simulink model "controller_final"  (R2024a)
settings: Solver=FixedStepAuto  StartTime=0.0  StopTime=10.0  FixedStep=1/100  RelTol=1e-3
settings Model: Creator=DAUIN-Win10  LastModifiedBy=mahdy
settings OptimizationCC: ReuseModelBlockBuffer=off
settings DebuggingCC: UnconnectedInputMsg=warning  UnconnectedOutputMsg=warning  UnconnectedLineMsg=warning
settings ModelReferenceCC: EnableRefExpFcnMdlSchedulingChecks=on
settings RTWCC: GPUComputeCapability=3.5  DLArmComputeVersion=19.05

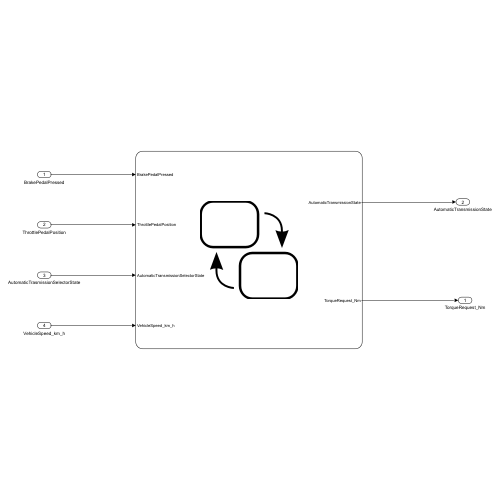
[thumbnail: Simulink's stored preview of the top-level diagram]
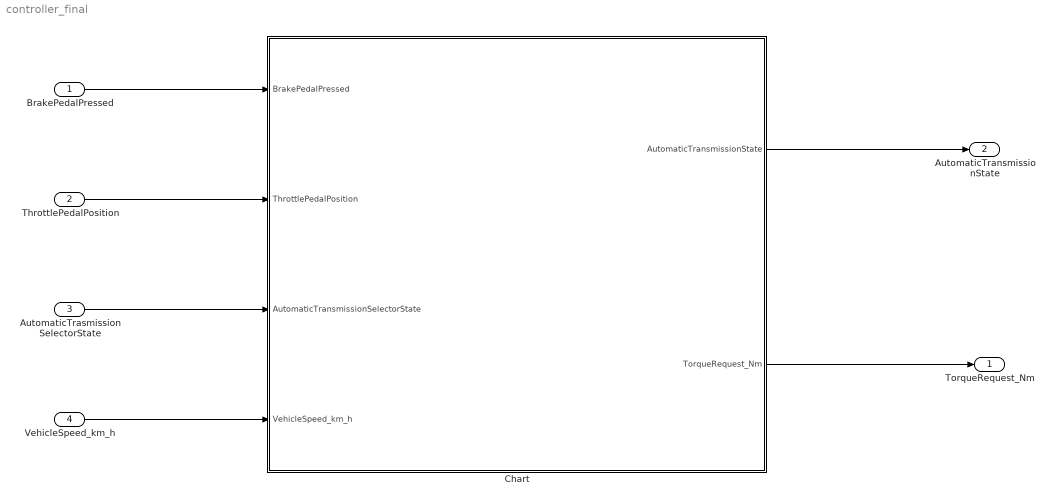
== system controller_final ==
  BrakePedalPressed : Inport  OutDataTypeStr=boolean
  ThrottlePedalPosition : Inport  Port=2  OutDataTypeStr=single
  AutomaticTrasmissionSelectorState : Inport  Port=3  OutDataTypeStr=Enum: TransmissionState
  VehicleSpeed_km_h : Inport  Port=4  OutDataTypeStr=single  Unit=km/h
  Chart : Stateflow chart  TreatAsAtomicUnit=on
  TorqueRequest_Nm : Outport  OutDataTypeStr=single  Unit=N*m
  AutomaticTransmissionState : Outport  Port=2  OutDataTypeStr=Enum: TransmissionState
  wires:
  VehicleSpeed_km_h/1 -> Chart/4(VehicleSpeed_km_h)
  AutomaticTrasmissionSelectorState/1 -> Chart/3(AutomaticTransmissionSelectorState)
  ThrottlePedalPosition/1 -> Chart/2(ThrottlePedalPosition)
  BrakePedalPressed/1 -> Chart/1(BrakePedalPressed)
  Chart/1(AutomaticTransmissionState) -> AutomaticTransmissionState/1
  Chart/2(TorqueRequest_Nm) -> TorqueRequest_Nm/1

== stateflow chart controller_final/Chart ==
  state Reverse
    entry:
    AutomaticTransmissionState =TransmissionState. Reverse;
    during:
    TorqueRequest_Nm = -ThrottlePedalPosition*MAX_TORQUE_REVERSE;
  state Park
    entry:
    AutomaticTransmissionState = TransmissionState.Park;
    TorqueRequest_Nm = 0;
  state Neutral
    entry:
    AutomaticTransmissionState = TransmissionState.Neutral;
    TorqueRequest_Nm = 0;
  state Bmode
    entry:
    AutomaticTransmissionState = TransmissionState.Brake;
    state Regenerative_Braking
      during:
      TorqueRequest_Nm =- MAX_TORQUE*(1-3*ThrottlePedalPosition)
    state Acceleration
      during:
      TorqueRequest_Nm =MAX_TORQUE*(ThrottlePedalPosition-1/3)*3/2;
    state Stop
      entry:
      TorqueRequest_Nm = 0;
    Acceleration -> Regenerative_Braking : [ThrottlePedalPosition<=1/3]
    Regenerative_Braking -> Acceleration [order 1] : [ThrottlePedalPosition>1/3]
    Stop -> Acceleration : [ThrottlePedalPosition>1/3]
    Regenerative_Braking -> Stop [order 2] : [ 0<ThrottlePedalPosition<=1/3 &&VehicleSpeed_km_h<=0.05 ]
    (default) -> Stop
  state Drive
    entry:
    AutomaticTransmissionState = TransmissionState.Drive;
    during:
    TorqueRequest_Nm = ThrottlePedalPosition*MAX_TORQUE;
  Reverse -> Neutral : [AutomaticTransmissionSelectorState ==TransmissionState. Neutral || AutomaticTransmissionSelectorState ==TransmissionState. Drive ||AutomaticTransmissionSelectorState ==TransmissionState. Brake||AutomaticTransmissionSelectorState ==TransmissionState. Park]
  Neutral -> Reverse [order 3] : [ VehicleSpeed_km_h<5 && AutomaticTransmissionSelectorState ==TransmissionState. Reverse &&BrakePedalPressed ==1]
  (default) -> Park
  Neutral -> Park [order 2] : [BrakePedalPressed ==1 && abs(VehicleSpeed_km_h)<5 && AutomaticTransmissionSelectorState == TransmissionState.Park]
  Park -> Neutral : [BrakePedalPressed ==1 && (AutomaticTransmissionSelectorState == TransmissionState.Reverse||AutomaticTransmissionSelectorState == TransmissionState.Neutral || AutomaticTransmissionSelectorState==TransmissionState.Brake|| AutomaticTransmissionSelectorState == TransmissionState.Drive)]
  Drive -> Neutral [order 1] : [AutomaticTransmissionSelectorState ==TransmissionState. Neutral||AutomaticTransmissionSelectorState == TransmissionState.Reverse||AutomaticTransmissionSelectorState == TransmissionState.Park]
  Neutral -> Drive [order 1] : [BrakePedalPressed==1 && VehicleSpeed_km_h>-5 && AutomaticTransmissionSelectorState ==TransmissionState. Drive || AutomaticTransmissionSelectorState == TransmissionState.Brake ]
  Drive -> Bmode [order 2] : [AutomaticTransmissionSelectorState == TransmissionState.Brake ]
  Bmode -> Drive : [AutomaticTransmissionSelectorState == TransmissionState.Drive||AutomaticTransmissionSelectorState == TransmissionState.Neutral||AutomaticTransmissionSelectorState == TransmissionState.Reverse||AutomaticTransmissionSelectorState == TransmissionState.Park]
  data: BrakePedalPressed input boolean; ThrottlePedalPosition input single; AutomaticTransmissionSelectorState input Enum: TransmissionState; VehicleSpeed_km_h input single; AutomaticTransmissionState output Enum: TransmissionState; TorqueRequest_Nm output single; MAX_TORQUE_REVERSE local =40; MAX_TORQUE local =80
